simulink model "MCP_phase3_fullobsv"  (R2020a)
settings: Solver=VariableStepAuto  StartTime=0.0  StopTime=10.0  RelTol=1e-3
settings Model: Creator=rafiee  LastModifiedBy=Lenovo
settings DataIOCC: ReturnWorkspaceOutputs=off
settings DebuggingCC: ArithmeticOperatorsInVariantConditions=warning
settings SFSimCC: SimUseLocalCustomCode=off  CustomCodeUndefinedFunction=UseInterfaceOnly
settings RTWCC: RTWUseLocalCustomCode=off
settings CodeAppCC: StateflowObjectComments=on

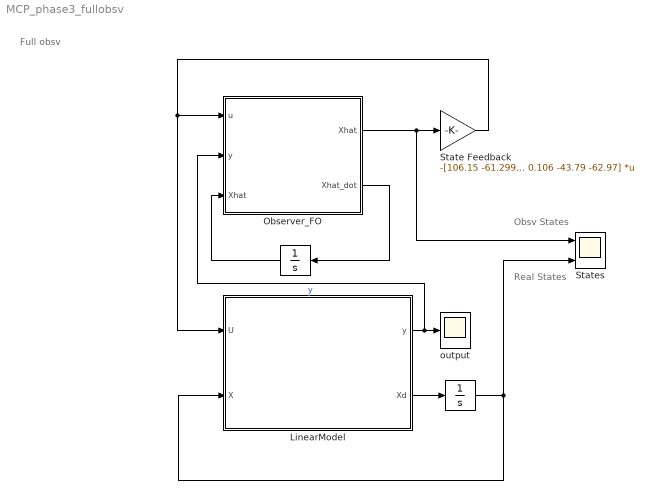
== system MCP_phase3_fullobsv ==
  note: Real States
  note: Obsv States
  note: Full obsv
  " " : Integrator  InitialCondition=[0;2;1;1;0;0]
  "  " : Integrator  InitialCondition=[0;0;0;0;0;0]
  LinearModel : MATLAB Function  TreatAsAtomicUnit=on
  Observer_FO : MATLAB Function  TreatAsAtomicUnit=on
  State Feedback : Gain  Gain=-[106.15 -61.299 0.111 0.986 160.72 57.96; 169.55 189.92 1.35 0.106 -43.79 -62.97]  Multiplication=Matrix(K*u)
  States : Scope  NumInputPorts=2
  "output " : Scope
  wires:
  LinearModel/2(Xd) -> " "/1
  LinearModel/1(y) -> Observer_FO/2(y), "output "/1  "y"
  "  "/1 -> Observer_FO/3("Xhat ")
  Observer_FO/2(Xhat_dot) -> "  "/1
  State Feedback/1 -> Observer_FO/1(u), LinearModel/1(U)
  Observer_FO/1(Xhat) -> States/1, State Feedback/1
  " "/1 -> States/2, LinearModel/2(X)

== matlab function MCP_phase3_fullobsv/Observer_FO ==
  data: Xhat output; u input; Xhat_dot output; y input; Xhat input
function [Xhat, Xhat_dot]= observer_FO(u, y, Xhat)

A = [ -0.0189,  0.029,      0, 0.00306,       0,       0;
       0, -0.029, 0.0065,       0,       0,       0;
       0,      0, -0.476,       0,       0,       0;
       0,      0,      0,    -0.5,       0,       0;
       0,      0, 0.0035,       0, -0.0191,  0.0349;
       0,      0,      0, 0.00714,       0, -0.0349];

B =[0,     0;
   0,     0;
   0, 0.476;
   0.5,     0;
   0,     0;
   0,     0];

C = [1.0, 0, 0, 0, 0, 0;
     0, 0, 0, 0, 1.0, 0];
 
L = [0.367, -0.0766;
      0.77,  -0.525;
    0.257,   -1.66;
 -0.00453,  0.0113;
  -0.0573,   0.655;
   -0.323,    2.12];

Xhat_dot = A*Xhat + B*u + L*(y - C*Xhat);

== matlab function MCP_phase3_fullobsv/LinearModel ==
  data: y output; U input; X input; Xd output
function [y, Xd]  = linear_plant(U, X)

A = [ -0.0189,  0.029,      0, 0.00306,       0,       0;
       0, -0.029, 0.0065,       0,       0,       0;
       0,      0, -0.476,       0,       0,       0;
       0,      0,      0,    -0.5,       0,       0;
       0,      0, 0.0035,       0, -0.0191,  0.0349;
       0,      0,      0, 0.00714,       0, -0.0349];

B =[0,     0;
   0,     0;
   0, 0.476;
   0.5,     0;
   0,     0;
   0,     0];

C = [1.0, 0, 0, 0, 0, 0;
     0, 0, 0, 0, 1.0, 0];
Xd = A * X + B * U; 
y = C*X;
